simulink model "HBridgeLut"  (R2025a)
settings: Solver=VariableStepAuto  StartTime=0.0  StopTime=10.0  RelTol=1e-3
undefined symbols (not defined in the file): TTL_on, Va_batt
libraries: simulink x2
settings Model: DataDictionary=Hbridge.sldd  Creator=tecnicomcbti  LastModifiedBy=tecnicomcbti

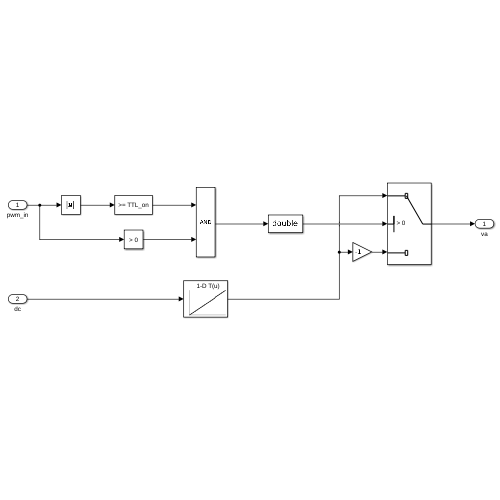
[thumbnail: Simulink's stored preview of the top-level diagram]
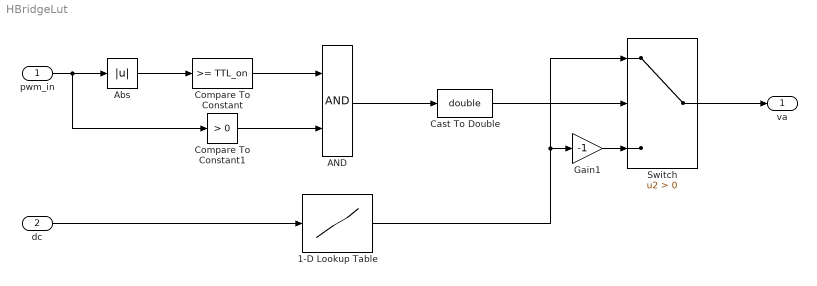
== system HBridgeLut ==
  pwm_in : Inport
  dc : Inport  Port=2
  1-D Lookup Table : Lookup_n-D  NumberOfTableDimensions=1  BreakpointsForDimension1=linspace(0,1,20)  Table=Va_batt.*linspace(0,1,20)  InternalRulePriority=Speed  RndMeth=Simplest
  AND : Logic  AllPortsSameDT=off  OutDataTypeStr=boolean
  Abs : Abs  SaturateOnIntegerOverflow=off
  Cast To Double : DataTypeConversion  OutDataTypeStr=double  SaturateOnIntegerOverflow=off  RndMeth=Floor
  Compare To Constant : simulink/Logic and Bit Operations/Compare To Constant  relop=>=  const=TTL_on  OutDataTypeStr=boolean
  Compare To Constant1 : simulink/Logic and Bit Operations/Compare To Constant  relop=>  const=0  OutDataTypeStr=boolean
  Gain1 : Gain  Gain=-1
  Switch : Switch  Criteria=u2 > Threshold  SaturateOnIntegerOverflow=off  InputSameDT=off
  va : Outport
  wires:
  pwm_in/1 -> Compare To Constant1/1, Abs/1
  Abs/1 -> Compare To Constant/1
  Compare To Constant/1 -> AND/1
  Compare To Constant1/1 -> AND/2
  dc/1 -> 1-D Lookup Table/1
  AND/1 -> Cast To Double/1
  Cast To Double/1 -> Switch/2
  1-D Lookup Table/1 -> Switch/1, Gain1/1
  Switch/1 -> va/1
  Gain1/1 -> Switch/3
